simulink model "EX4_ex2"  (R2018b)
settings: Solver=VariableStepAuto  StartTime=0.0  StopTime=2  RelTol=1e-3
settings Model: Creator=吳俊逸  LastModifiedBy=吳俊逸

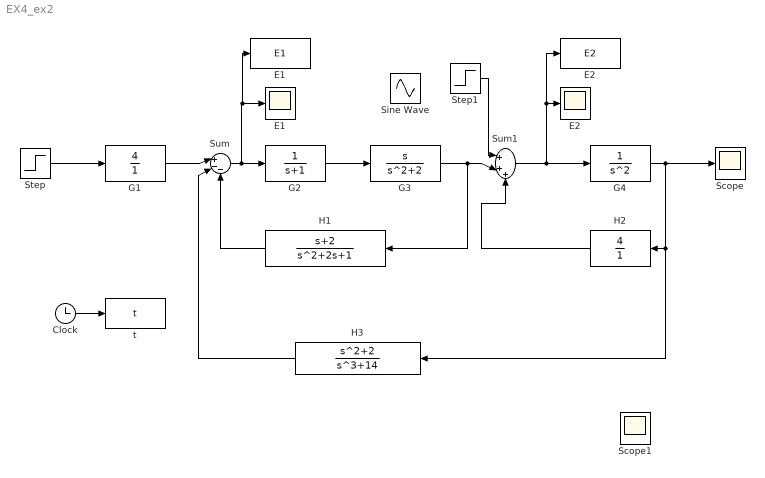
== system EX4_ex2 ==
  Clock : Clock
  E1 : Scope
  "E1 " : ToWorkspace  VariableName=E1  SampleTime=-1
  E2 : Scope
  "E2 " : ToWorkspace  VariableName=E2  SampleTime=-1
  "G1 " : TransferFcn  Numerator=[4]  Denominator=[1]
  G2 : TransferFcn  Denominator=[1 1]
  G3 : TransferFcn  Numerator=[1 0]  Denominator=[1 0 2]
  G4 : TransferFcn  Denominator=[1 0 0]
  H1 : TransferFcn  Numerator=[1 2]
  H2 : TransferFcn  Numerator=[4]  Denominator=[1]
  H3 : TransferFcn  Numerator=[1 0 2 ]  Denominator=[1 0 0 14]
  Scope : Scope
  Scope1 : Scope
  Sine Wave : Sin  Amplitude=0.1  SampleTime=0
  Step : Step  Time=0  SampleTime=0
  Step1 : Step  Time=0  After=0.1  SampleTime=0
  Sum : Sum  Inputs=|+--
  Sum1 : Sum  Inputs=|+++
  "t " : ToWorkspace  VariableName=t  SampleTime=-1
  wires:
  "G1 "/1 -> Sum/1
  Sum/1 -> "E1 "/1, E1/1, G2/1
  H1/1 -> Sum/3
  H3/1 -> Sum/2
  G2/1 -> G3/1
  G3/1 -> Sum1/2, H1/1
  G4/1 -> Scope/1, H3/1, H2/1
  Sum1/1 -> "E2 "/1, E2/1, G4/1
  H2/1 -> Sum1/3
  Step/1 -> "G1 "/1
  Clock/1 -> "t "/1
  Step1/1 -> Sum1/1
